simulink model "TwoSwitchForward"  (R2018a)
settings: Solver=VariableStepAuto  StartTime=0.0  StopTime=10.0  RelTol=1e-3
undefined symbols (not defined in the file): Lm
libraries: powerlib x19, powerlib_meascontrol x1
settings Model: Creator=user  LastModifiedBy=user

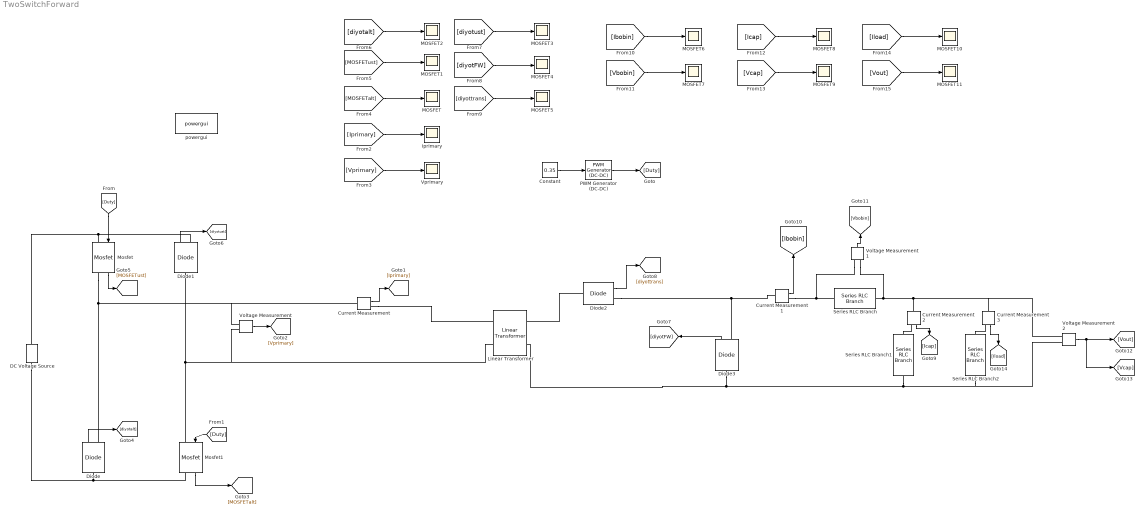
== system TwoSwitchForward ==
  Constant : Constant  Value=0.35
  Current Measurement{,1..3} (4 alike) : powerlib/Measurements/Current Measurement  PhasorSimulation=off  OutputType=Complex  PSBequivalent=0
  DC Voltage Source : powerlib/Electrical Sources/DC Voltage Source  Amplitude=100  Measurements=None
  Diode{,1..3} (4 alike) : powerlib/Power Electronics/Diode  Ron=0.001  Lon=0  Vf=0.8  IC=0  UseSnubber=0  Rs=500  Cs=250e-9  Measurements=on
  Iprimary : Scope
  Linear Transformer : powerlib/Elements/Linear Transformer  UNITS=pu  NominalPower=[ 250e6 40000 ]  winding1="[ 735e3  0.002  0.08 ]"  winding2="[ 315e3  0.002  0.08 ]"  ThreeWindings=off  winding3=[ 315e3 0.002 0.08 ]  RmLm=[ 500 Lm]  Measurements=None  DataType=off
  MOSFET{,1..11} (12 alike) : Scope
  Mosfet : powerlib/Power Electronics/Mosfet  Ron=0.1  Lon=0  Rd=0.01  Vfd=0  IC=0  Rs=1e5  Cs=inf  Measurements=on
  Mosfet1 : powerlib/Power Electronics/Mosfet  Ron=0.1  Lon=0  Rd=0.01  Vfd=0  IC=0  Rs=1e5  Cs=inf  Measurements=on
  PWM Generator (DC-DC) : powerlib_meascontrol/Pulse & Signal Generators/PWM Generator (DC-DC)  Fsw=40000  Ts=0
  Series RLC Branch : powerlib/Elements/Series RLC Branch  LConnTagsString=__new0  RConnTagsString=__new0  BranchType=L  Resistance=1  Inductance=1  SetiL0=off  InitialCurrent=0  Capacitance=1e-6  Setx0=off  InitialVoltage=0  Measurements=None
  Series RLC Branch1 : powerlib/Elements/Series RLC Branch  LConnTagsString=__new0  RConnTagsString=__new0  BranchType=C  Resistance=1  Inductance=1e-3  SetiL0=off  InitialCurrent=0  Capacitance=1e-6  Setx0=off  InitialVoltage=0  Measurements=None
  Series RLC Branch2 : powerlib/Elements/Series RLC Branch  LConnTagsString=__new0  RConnTagsString=__new0  BranchType=R  Resistance=1  Inductance=1e-3  SetiL0=off  InitialCurrent=0  Capacitance=1e-6  Setx0=off  InitialVoltage=0  Measurements=None
  Voltage Measurement : powerlib/Measurements/Voltage Measurement  PhasorSimulation=off  OutputType=Complex  PSBequivalent=0
  Voltage Measurement1 : powerlib/Measurements/Voltage Measurement  PhasorSimulation=off  OutputType=Complex  PSBequivalent=0
  Voltage Measurement2 : powerlib/Measurements/Voltage Measurement  PhasorSimulation=off  OutputType=Complex  PSBequivalent=0
  Vprimary : Scope
  powergui : powerlib/powergui  Priority=1  SimulationMode=Continuous  SampleTime=50e-6  frequency=60  Iterations=50  frequencyindice=0  Pbase=100e6  ErrMax=1e-4  UnitsV=kV  UnitsW=MW  buscounter=0  FunctionMessages=off  echomessages=off  EnableUseOfTLC=off  CurrentSourceSwitches=off  DisableSnubberDevices=off  DisableRonSwitches=off  DisableVfSwitches=off  DisplayEquations=off  SolverType=Tustin/Backward Euler (TBE)  Interpol=off  ExternalGateDelay=off  methode=off  Ts=100  x0status=blocks  SPID=on  SwTol=0  HookPort=off  RestoreLinks=warning  ResistiveCurrentMeasurement=off  Frange=[0:2:500]  Ylog=off  Xlog=on  ShowGrid=off  save=off  variable=ZData  structure=0  ZoomFFT=off  StartTime=0.0  cycles=1  DisplayStyle=1  fundamental=60  FreqAxis=off  MaxFrequency=1000  frequencyindicesteady=1  RmsSteady=1  display=off
  wires:
  Constant/1 -> PWM Generator (DC-DC)/1
  PWM Generator (DC-DC)/1 -> [Duty]
  [Duty] -> Mosfet1/1
  [Duty] -> Mosfet/1
  Current Measurement/1 -> [Iprimary]
  [Iprimary] -> Iprimary/1
  Voltage Measurement/1 -> [Vprimary]
  [Vprimary] -> Vprimary/1
  Mosfet1/1 -> [MOSFETalt]
  [MOSFETalt] -> MOSFET/1
  Diode/1 -> [diyotalt]
  [MOSFETust] -> MOSFET1/1
  Mosfet/1 -> [MOSFETust]
  [diyotalt] -> MOSFET2/1
  Diode1/1 -> [diyotust]
  [diyotust] -> MOSFET3/1
  Diode3/1 -> [diyotFW]
  [diyotFW] -> MOSFET4/1
  [diyottrans] -> MOSFET5/1
  Diode2/1 -> [diyottrans]
  Current Measurement2/1 -> [Icap]
  Current Measurement1/1 -> [Ibobin]
  Voltage Measurement1/1 -> [Vbobin]
  Voltage Measurement2/1 -> [Vcap], [Vout]
  Current Measurement3/1 -> [Iload]
  [Ibobin] -> MOSFET6/1
  [Vbobin] -> MOSFET7/1
  [Icap] -> MOSFET8/1
  [Vcap] -> MOSFET9/1
  [Iload] -> MOSFET10/1
  [Vout] -> MOSFET11/1
  connections:
  DC Voltage Source/RConn1 -- Diode1/RConn1 -- Mosfet/LConn1
  Mosfet/RConn1 -- Voltage Measurement/LConn1 -- Current Measurement/LConn1 -- Diode/RConn1
  DC Voltage Source/LConn1 -- Mosfet1/RConn1 -- Diode/LConn1
  Mosfet1/LConn1 -- Voltage Measurement/LConn2 -- Linear Transformer/LConn2 -- Diode1/LConn1
  Diode3/LConn1 -- Voltage Measurement2/LConn2 -- Series RLC Branch2/RConn1 -- Series RLC Branch1/RConn1 -- Linear Transformer/RConn2
  Diode2/LConn1 -- Linear Transformer/RConn1
  Diode2/RConn1 -- Current Measurement1/LConn1 -- Diode3/RConn1
  Series RLC Branch/RConn1 -- Current Measurement3/LConn1 -- Voltage Measurement2/LConn1 -- Current Measurement2/LConn1 -- Voltage Measurement1/LConn2
  Current Measurement/RConn1 -- Linear Transformer/LConn1
  Current Measurement1/RConn1 -- Voltage Measurement1/LConn1 -- Series RLC Branch/LConn1
  Current Measurement2/RConn1 -- Series RLC Branch1/LConn1
  Current Measurement3/RConn1 -- Series RLC Branch2/LConn1
